simulink subsystem "Gravity_and_Propulsion"  (R2024b)
settings: Solver=VariableStepAuto  StartTime=0.0  StopTime=10.0  RelTol=1e-3
undefined symbols (not defined in the file or in its folder): engine_thrust_factor, F_thrust, mass, sim_time
settings Model: Creator=joedo  LastModifiedBy=finnb

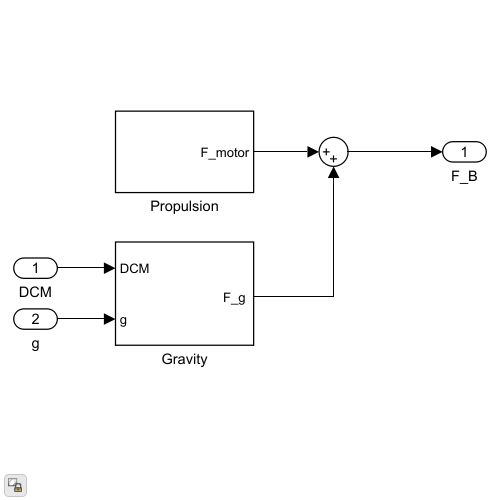
[thumbnail: Simulink's stored preview of the top-level diagram]
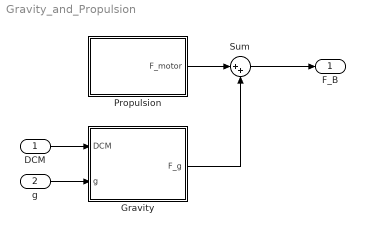
== system Gravity_and_Propulsion ==
  DCM : Inport
  g : Inport  Port=2
  "Gravity " : Subsystem
  "Propulsion " : Subsystem
  Sum : Sum  Inputs=|++
  F_B : Outport  VectorParamsAs1DForOutWhenUnconnected=off
  wires:
  Sum/1 -> F_B/1
  "Propulsion "/1(F_motor) -> Sum/1
  DCM/1 -> "Gravity "/1(DCM)
  "Gravity "/1("F_g ") -> Sum/2
  g/1 -> "Gravity "/2(g)

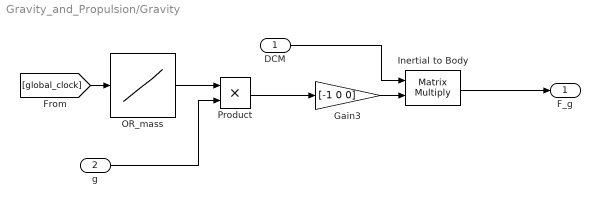
== system Gravity_and_Propulsion/Gravity  ==
  DCM : Inport
  g : Inport  Port=2
  Gain3 : Gain  Gain=[-1 0 0]
  Inertial to Body : Product  Multiplication=Matrix(*)  InputSameDT=on  SaturateOnIntegerOverflow=on  OutDataTypeStr=Inherit: Same as first input
  OR_mass : Lookup_n-D  NumberOfTableDimensions=1  BreakpointsForDimension1=sim_time  Table=mass  InternalRulePriority=Speed  RndMeth=Simplest
  Product : Product
  "F_g " : Outport  VectorParamsAs1DForOutWhenUnconnected=off
  wires:
  [global_clock] -> OR_mass/1
  g/1 -> Product/2
  Product/1 -> Gain3/1
  OR_mass/1 -> Product/1
  Gain3/1 -> Inertial to Body/2
  DCM/1 -> Inertial to Body/1
  Inertial to Body/1 -> "F_g "/1

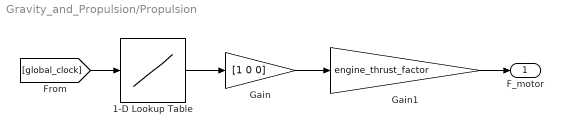
== system Gravity_and_Propulsion/Propulsion  ==
  1-D Lookup Table : Lookup_n-D  NumberOfTableDimensions=1  BreakpointsForDimension1=sim_time  Table=F_thrust  InternalRulePriority=Speed  RndMeth=Simplest
  Gain : Gain  Gain=[1 0 0]
  Gain1 : Gain  Gain=engine_thrust_factor
  F_motor : Outport  VectorParamsAs1DForOutWhenUnconnected=off
  wires:
  Gain1/1 -> F_motor/1
  [global_clock] -> 1-D Lookup Table/1
  Gain/1 -> Gain1/1
  1-D Lookup Table/1 -> Gain/1
